simulink library "FuelSystemLibrary"  (R2014b)
settings: Solver=ode45  SolverMode=SingleTasking  StartTime=0.0  StopTime=10.0  RelTol=1e-3
undefined symbols (not defined in the file): BooleanOff, BooleanOn, BoolThreshold, BowserOnPressure, CouplingOffPressure, CouplingOnPressure, DefaultTemp, DiffuserResistance, DiscreteSwitchOff, DiscreteSwitchOn, DiscreteSwitchThreshold, FloatingPressure, FlowNoOverride, FspSamplingPeriod, FuelSpecificHeatCapacity, g, InfiniteFlow, InfiniteMass, InfiniteResistance, InfiniteTime, InfiniteVolume, kpl2kpm3, MaxAValue, MaxBValue, MeterNoReset, MinAValue, MinBValue, NearZeroMass, NearZeroTime, NoError, NominalAValue, NominalBValue, NonRetResistance, NoReset, NullBasePress, PerCycle2PerSec, PerSec2PerCycle, PipeDisconnected, PipeResistance, PumpOnTime, TankFixedMassError, TankInletResistance, TankInstPortStartOffset, TankNoReset, TypicalFuelDensity, ValveClosedPosition, ValveOnResistance, ValveOpenPosition, ValveOpenTime
libraries: FuelSystemLibrary x251, WrightSolverLib x50, simulink x1
(part 1 of 4)
settings Model: ExtModeAutoUpdateStatusClock=off  Creator=SWright2  LastModifiedBy=sj3-wright

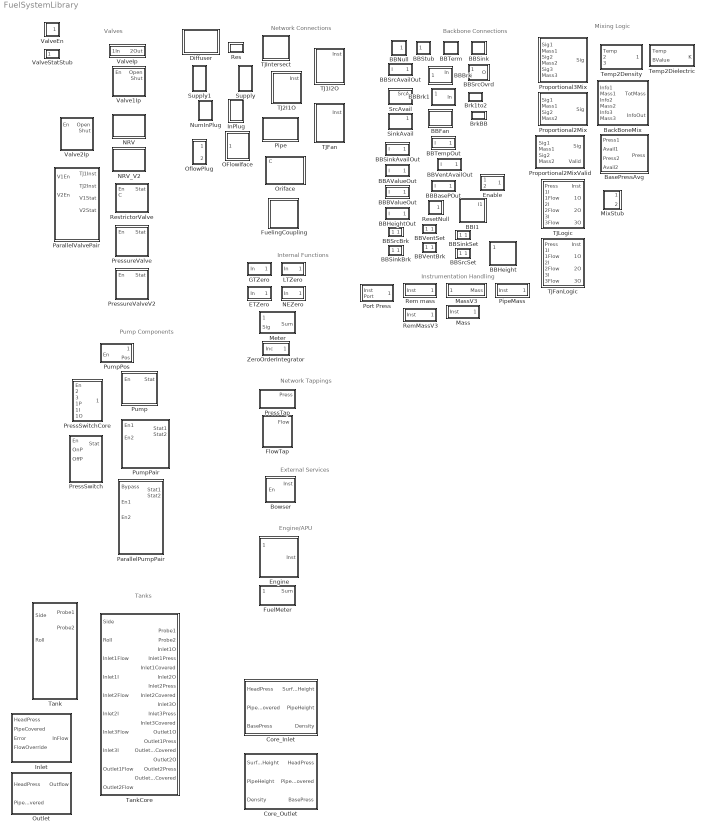
== system FuelSystemLibrary ==
  note: Network Tappings
  note: Network Connections
  note: Valves
  note: Internal Functions
  note: Mixing Logic
  note: External Services
  note: Pump Components
  note: Tanks
  note: Engine/APU
  note: Backbone Connections
  note: Instrumentation Handling
  BBAValueOut : Subsystem
  BBBValueOut : Subsystem
  BBBasePOut : Subsystem
  BBBrk : Subsystem
  BBBrk1 : Subsystem
  BBFan : Subsystem
  BBHeight : Subsystem
  BBHeightOut : Subsystem
  BBI1 : Subsystem
  BBNull : Subsystem
  BBSink : Subsystem
  BBSinkAvailOut : Subsystem
  BBSinkBrk : Subsystem
  BBSinkSet : Subsystem
  BBSrcAvailOut : Subsystem
  BBSrcBrk : Subsystem
  BBSrcOvrd : Subsystem
  BBSrcSet : Subsystem
  BBStub : Subsystem
  BBTempOut : Subsystem
  BBTerm : Subsystem
  BBVentAvailOut : Subsystem
  BBVentBrk : Subsystem
  BBVentSet : Subsystem
  BackBoneMix : Subsystem  RTWFcnName=BackBoneMix  RTWFileName=BackBoneMix
      settings: RTWFcnNameOpts=User specified  RTWFileNameOpts=User specified
  BasePressAvg : Subsystem
  Bowser : Subsystem
  Brk1to2 : Subsystem
  BrkBB : Subsystem
  Core_Inlet : Subsystem
  Core_Outlet : Subsystem
  Diffuser : Subsystem
  ETZero : Subsystem
  Enable : Subsystem
  Engine : Subsystem
  FlowTap : Subsystem
  FuelMeter : Subsystem
  FuelingCoupling : Subsystem
  GTZero : Subsystem  TreatAsAtomicUnit=on
  InPlug : Subsystem
  Inlet : Subsystem  mask{TankInletResistance=TankInletResistance}
      mask init:
      | InfiniteResistance = -999.0;
  LTZero : Subsystem  TreatAsAtomicUnit=on
  Mass : Subsystem
  MassV3 : Subsystem
  Meter : Subsystem  TreatAsAtomicUnit=on  RTWFcnName=Meter  RTWFileName=Meter
      settings: RTWFcnNameOpts=User specified  RTWFileNameOpts=User specified
  MixStub : Subsystem
  NEZero : Subsystem  TreatAsAtomicUnit=on
  NRV : Subsystem
  NRV_V2 : Subsystem
  NumInPlug : Subsystem
  OFlowIface : Subsystem
  OflowPlug : Subsystem
  Oriface : Subsystem
  Outlet : Subsystem
  ParallelPumpPair : Subsystem
  ParallelValvePair : Subsystem
  Pipe : Subsystem
  PipeMass : Subsystem
  Port Press : Subsystem  TreatAsAtomicUnit=on  RTWFcnName=PortPressure  RTWFileName=PortPressure
      settings: RTWFcnNameOpts=User specified  RTWFileNameOpts=User specified
  PressSwitch : Subsystem
  PressSwitchCore : Subsystem  TreatAsAtomicUnit=on  RTWFcnName=PressSwitchCore  RTWFileName=PressSwitchCore
      settings: RTWFcnNameOpts=User specified  RTWFileNameOpts=User specified
  PressTap : Subsystem
  PressureValve : Subsystem
  PressureValveV2 : Subsystem
  Proportional2Mix : Subsystem  RTWFcnName=Proportional2Mix  RTWFileName=Proportional2Mix
      settings: RTWFcnNameOpts=User specified  RTWFileNameOpts=User specified
  Proportional2MixValid : Subsystem  RTWFcnName=Proportional2MixValid  RTWFileName=Proportional2MixValid
      settings: RTWFcnNameOpts=User specified  RTWFileNameOpts=User specified
  Proportional3Mix : Subsystem  RTWFcnName=Proportional3Mix  RTWFileName=Proportional3Mix
      settings: RTWFcnNameOpts=User specified  RTWFileNameOpts=User specified
  Pump : Subsystem
  PumpPair : Subsystem
  PumpPos : Subsystem  TreatAsAtomicUnit=on
  Rem mass : Subsystem
  RemMassV3 : Subsystem
  Res : Subsystem
  ResetNull : Subsystem
  RestrictorValve : Subsystem
  SinkAvail : Subsystem
  SrcAvail : Subsystem
  Supply : Subsystem
  Supply1 : Subsystem
  TJ1I2O : Subsystem
  TJ2I1O : Subsystem
  TJFan : Subsystem
  TJFanLogic : Subsystem
  TJIntersect : Subsystem
  TJLogic : Subsystem
  Tank : Subsystem
  TankCore : Subsystem
      settings: RTWSystemCode=Nonreusable function
  Temp2Density : Subsystem  TreatAsAtomicUnit=on  RTWFcnName=Temp2Density  RTWFileName=Temp2Density
      settings: RTWFcnNameOpts=User specified  RTWFileNameOpts=User specified
  Temp2Dielectric : Subsystem  TreatAsAtomicUnit=on  RTWFcnName=Temp2Dielectric  RTWFileName=Temp2Dielectric
      settings: RTWFcnNameOpts=User specified  RTWFileNameOpts=User specified
  Valve1Ip : Subsystem
  Valve2Ip : Subsystem
  ValveEn : Subsystem  TreatAsAtomicUnit=on  RTWFcnName=ValveEn
      settings: RTWFcnNameOpts=User specified
  ValveIp : Subsystem
  ValveStatStub : Subsystem
  ZeroOrderIntegrator : Subsystem  TreatAsAtomicUnit=on

== system FuelSystemLibrary/BBAValueOut ==
  note: BBAValueOut - Block to seperate Flow A Value form Backbone Network
      |
      | Revision History -
      | Issue 1.0 - ?? - SW - Initial Issue
      | Issue 1.1 - 28th October 2005 - DR - Added to FSP Generic Library
      | Issue 1.2 - 16th December 2008 - SW - SinkAvailable added
  I : Inport
  Demux1 : Demux  Outputs=[1 1 1 1 1 1 1 1]
  Terminator{1..7} (7 alike) : Terminator
  AVal : Outport
  wires:
  I/1 -> Demux1/1
  Demux1/5 -> Terminator6/1  "SrcAvailable"
  Demux1/2 -> Terminator4/1  "Temp"
  Demux1/1 -> Terminator3/1  "BasePress"
  Demux1/3 -> AVal/1  "AValue"
  Demux1/4 -> Terminator5/1  "BValue"
  Demux1/6 -> Terminator1/1  "SinkAvailable"
  Demux1/7 -> Terminator2/1  "VentAvailable"
  Demux1/8 -> Terminator7/1  "Height"

== system FuelSystemLibrary/BBBValueOut ==
  note: BBBValueOut - Block to seperate Flow B Value form Backbone Network
      |
      | Revision History -
      | Issue 1.0 - ?? - SW - Initial Issue
      | Issue 1.1 - 28th October 2005 - DR - Added to FSP Generic Library
      | Issue 1.2 - 16th December 2008 - SW - SinkAvailable added
  I : Inport
  Demux1 : Demux  Outputs=[1 1 1 1 1 1 1 1]
  Terminator{1..7} (7 alike) : Terminator
  BVal : Outport
  wires:
  I/1 -> Demux1/1
  Demux1/5 -> Terminator6/1  "SrcAvailable"
  Demux1/2 -> Terminator4/1  "Temp"
  Demux1/1 -> Terminator3/1  "BasePress"
  Demux1/3 -> Terminator5/1  "AValue"
  Demux1/4 -> BVal/1  "BValue"
  Demux1/6 -> Terminator1/1  "SinkAvailable"
  Demux1/7 -> Terminator2/1  "VentAvailable"
  Demux1/8 -> Terminator7/1  "Height"

== system FuelSystemLibrary/BBBasePOut ==
  note: BBBasePOut - Block to seperate Base Pressure
      | signal from the Backbone Network
      |
      | Revision History -
      | Issue 1.0 - ?? - SW - Initial Issue
      | Issue 1.1 - 28th October 2005 - DR - Added to FSP Generic Library
      | Issue 1.2 - 16th December 2008 - SW - SinkAvailable added
  I : Inport
  Demux1 : Demux  Outputs=[1 1 1 1 1 1 1 1]
  Terminator{1..7} (7 alike) : Terminator
  Press : Outport
  wires:
  I/1 -> Demux1/1
  Demux1/2 -> Terminator3/1  "Temp"
  Demux1/1 -> Press/1  "BasePress"
  Demux1/3 -> Terminator5/1  "AValue"
  Demux1/4 -> Terminator4/1  "BValue"
  Demux1/5 -> Terminator1/1  "SrcAvailable"
  Demux1/6 -> Terminator2/1  "SinkAvailable"
  Demux1/7 -> Terminator6/1  "VentAvailable"
  Demux1/8 -> Terminator7/1  "Height"

== system FuelSystemLibrary/BBBrk ==
  In : Inport
  Two-Way Connection1 : TwoWayConnection
  BB : PMIOPort  Tag=PMCPort  Port=1  Side=Left
  Out : Outport
  wires:
  Two-Way Connection1/1 -> Out/1
  In/1 -> Two-Way Connection1/1
  connections:
  BB/RConn1 -- Two-Way Connection1/RConn1

== system FuelSystemLibrary/BBBrk1 ==
  In : Inport
  Two-Way Connection1 : TwoWayConnection
  BB : PMIOPort  Tag=PMCPort  Port=1  Side=Right
  Out : Outport
  wires:
  In/1 -> Two-Way Connection1/1
  Two-Way Connection1/1 -> Out/1
  connections:
  BB/RConn1 -- Two-Way Connection1/RConn1

== system FuelSystemLibrary/BBFan ==
  BBBrk1 : FuelSystemLibrary/BBBrk1
  BBBrk2 : FuelSystemLibrary/BBBrk1
  BBBrk3 : FuelSystemLibrary/BBBrk1
  BBNull : FuelSystemLibrary/BBNull
  BBStub : FuelSystemLibrary/BBStub
  BBStub1 : FuelSystemLibrary/BBStub
  In : PMIOPort  Tag=PMCPort  Port=1  Side=Left
  Out1 : PMIOPort  Tag=PMCPort  Port=2  Side=Right
  Out2 : PMIOPort  Tag=PMCPort  Port=3  Side=Right
  wires:
  BBBrk3/1 -> BBStub1/1
  BBBrk2/1 -> BBStub/1
  BBNull/1 -> BBBrk1/1
  BBBrk1/1 -> BBBrk3/1, BBBrk2/1
  connections:
  BBBrk3/RConn1 -- Out2/RConn1
  BBBrk2/RConn1 -- Out1/RConn1
  In/RConn1 -- BBBrk1/RConn1

== system FuelSystemLibrary/BBHeight ==
  note: Insert height at this point
  Height : Inport
  BBBrk : FuelSystemLibrary/BBBrk
  BBBrk1 : FuelSystemLibrary/BBBrk1
  Demux1 : Demux  Outputs=[1 1 1 1 1 1 1 1]
  Demux3 : Demux  Outputs=[1 1 1 1 1 1 1 1]
  Mux1 : Mux  Inputs=[1 1 1 1 1 1 1 1]
  Mux3 : Mux  Inputs=[1 1 1 1 1 1 1 1]
  Terminator : Terminator
  Terminator1 : Terminator
  BB1 : PMIOPort  Tag=PMCPort  Port=1  Side=Left
  BB2 : PMIOPort  Tag=PMCPort  Port=2  Side=Right
  wires:
  BBBrk/1 -> Demux1/1
  BBBrk1/1 -> Demux3/1
  [Height] -> Mux3/8
  Demux3/1 -> Mux3/1  "BasePress"
  Demux3/2 -> Mux3/2  "Temp"
  Demux3/3 -> Mux3/3  "AValue"
  Demux3/4 -> Mux3/4  "BValue"
  Demux3/5 -> Mux3/5  "SrcAvailable"
  Demux3/6 -> Mux3/6  "SinkAvailable"
  Demux3/8 -> Terminator/1  "Height"
  Demux3/7 -> Mux3/7  "VentAvailable"
  Mux3/1 -> BBBrk/1
  Demux1/1 -> Mux1/1  "BasePress"
  Demux1/2 -> Mux1/2  "Temp"
  Demux1/3 -> Mux1/3  "AValue"
  Demux1/4 -> Mux1/4  "BValue"
  Demux1/5 -> Mux1/5  "SrcAvailable"
  Demux1/6 -> Mux1/6  "SinkAvailable"
  Demux1/8 -> Terminator1/1  "Height"
  Demux1/7 -> Mux1/7  "VentAvailable"
  Height/1 -> [Height]
  [Height] -> Mux1/8
  Mux1/1 -> BBBrk1/1
  connections:
  BB1/RConn1 -- BBBrk1/RConn1
  BB2/RConn1 -- BBBrk/LConn1

== system FuelSystemLibrary/BBHeightOut ==
  note: BBHeightOut - Block to seperate Height Value form Backbone Network
      |
      | Revision History -
      | Issue 1.0 - 18th Mayt 2009 - SW - Initial Issue
  I : Inport
  Demux1 : Demux  Outputs=[1 1 1 1 1 1 1 1]
  Terminator{1..6,8} (7 alike) : Terminator
  Hght : Outport
  wires:
  I/1 -> Demux1/1
  Demux1/5 -> Terminator6/1  "SrcAvailable"
  Demux1/2 -> Terminator4/1  "Temp"
  Demux1/1 -> Terminator3/1  "BasePress"
  Demux1/3 -> Terminator5/1  "AValue"
  Demux1/4 -> Terminator8/1  "BValue"
  Demux1/6 -> Terminator1/1  "SinkAvailable"
  Demux1/7 -> Terminator2/1  "VentAvailable"
  Demux1/8 -> Hght/1  "Height"

== system FuelSystemLibrary/BBI1 ==
  note: Extract the inbound signal from port1
  BBBrk : FuelSystemLibrary/BBBrk
  BBBrk1 : FuelSystemLibrary/BBBrk1
  BB1 : PMIOPort  Tag=PMCPort  Port=1  Side=Left
  BB2 : PMIOPort  Tag=PMCPort  Port=2  Side=Right
  I1 : Outport
  wires:
  BBBrk1/1 -> I1/1, BBBrk/1
  BBBrk/1 -> BBBrk1/1
  connections:
  BB1/RConn1 -- BBBrk1/RConn1
  BBBrk/LConn1 -- BB2/RConn1

== system FuelSystemLibrary/BBNull ==
  note: BBNull
      |
      | Revision History -
      | Issue 1.0 - ?? - SW - Initial Issue
      | Issue 1.1 - 28th October 2005 - DR - Added to FSP Generic Library
      | Issue 1.2 - 7th July 2009 - SW - New elements added
  Constant1 : Constant  Value=DefaultTemp
  Constant{2,4..6} (4 alike) : Constant  Value=0
  Constant3 : Constant  Value=NullBasePress
  Constant8 : Constant  Value=NominalAValue
  Constant9 : Constant  Value=NominalBValue
  Mux : Mux  Inputs=[1 1 1 1 1 1 1 1]
  Nul : Outport
  wires:
  Constant1/1 -> Mux/2  "Temp"
  Constant3/1 -> Mux/1  "BasePress"
  Constant2/1 -> Mux/5  "SrcAvailable"
  Mux/1 -> Nul/1
  Constant8/1 -> Mux/3  "AValue"
  Constant9/1 -> Mux/4  "BValue"
  Constant4/1 -> Mux/6  "SinkAvailable"
  Constant5/1 -> Mux/7  "VentAvailable"
  Constant6/1 -> Mux/8  "Height"

== system FuelSystemLibrary/BBSink ==
  note: BBTerminator
      |
      | Revision History -
      | Issue 1.0 - 4th April 2011 - SW - Initial Issue
  BBBrk1 : FuelSystemLibrary/BBBrk
  BBBrk2 : FuelSystemLibrary/BBBrk1
  BBSinkSet : FuelSystemLibrary/BBSinkSet
  BBTerm : FuelSystemLibrary/BBTerm
  BB : PMIOPort  Tag=PMCPort  Port=1  Side=Left
  wires:
  BBBrk2/1 -> BBBrk1/1
  BBSinkSet/1 -> BBBrk2/1
  BBBrk1/1 -> BBSinkSet/1
  connections:
  BB/RConn1 -- BBBrk2/RConn1
  BBBrk1/LConn1 -- BBTerm/LConn1

== system FuelSystemLibrary/BBSinkAvailOut ==
  I : Inport
  Data Type Conversion : DataTypeConversion  OutDataTypeStr=double
  Demux : Demux  Outputs=[1 1 1 1 1 1 1 1]
  Terminator{1..7} (7 alike) : Terminator
  SinkA : Outport
  wires:
  Demux/6 -> Data Type Conversion/1  "SinkAvailable"
  Demux/4 -> Terminator5/1  "BValue"
  Demux/3 -> Terminator4/1  "AValue"
  Demux/1 -> Terminator2/1  "BasePress"
  Demux/2 -> Terminator3/1  "Temp"
  Demux/5 -> Terminator1/1  "SrcAvailable"
  I/1 -> Demux/1
  Demux/7 -> Terminator6/1  "VentAvailable"
  Demux/8 -> Terminator7/1  "Height"
  Data Type Conversion/1 -> SinkA/1

== system FuelSystemLibrary/BBSinkBrk ==
  note: Break Backbone Sink-Available Signal
  I : Inport
  Constant1 : Constant  Value=0
  Demux3 : Demux  Outputs=8
  Mux3 : Mux  Inputs=8
  Terminator : Terminator
  O : Outport
  wires:
  Demux3/1 -> Mux3/1  "BasePress"
  Demux3/2 -> Mux3/2  "Temp"
  Demux3/3 -> Mux3/3  "AValue"
  Demux3/4 -> Mux3/4  "BValue"
  Demux3/5 -> Mux3/5  "SrcAvailable"
  Constant1/1 -> Mux3/6
  Demux3/6 -> Terminator/1  "SinkAvailable"
  Demux3/8 -> Mux3/8  "Height"
  Demux3/7 -> Mux3/7  "VentAvailable"
  I/1 -> Demux3/1
  Mux3/1 -> O/1

== system FuelSystemLibrary/BBSinkSet ==
  note: Set Backbone Sink-Available Signal
  I : Inport
  Constant8 : Constant
  Demux2 : Demux  Outputs=8
  Mux3 : Mux  Inputs=8
  Terminator : Terminator
  O : Outport
  wires:
  Mux3/1 -> O/1
  Demux2/7 -> Mux3/7  "VentAvailable"
  Demux2/8 -> Mux3/8  "Height"
  Demux2/6 -> Terminator/1  "SinkAvailable"
  Demux2/5 -> Mux3/5  "SrcAvailable"
  Demux2/4 -> Mux3/4  "BValue"
  Demux2/3 -> Mux3/3  "AValue"
  Demux2/2 -> Mux3/2  "Temp"
  Demux2/1 -> Mux3/1  "BasePress"
  I/1 -> Demux2/1
  Constant8/1 -> Mux3/6

== system FuelSystemLibrary/BBSrcAvailOut ==
  note: BBFlowAvailOut - Block to seperate Flow
      | Available signal from the Backbone Network
      |
      | Revision History -
      | Issue 1.0 - ?? - SW - Initial Issue
      | Issue 1.1 - 28th October 2005 - DR - Added to FSP Generic Library
      | Issue 1.2 - 16th December 2008 - SW - SinkAvailable added
  I : Inport
  Data Type Conversion : DataTypeConversion  OutDataTypeStr=double
  Demux : Demux  Outputs=[1 1 1 1 1 1 1 1]
  Terminator{1..7} (7 alike) : Terminator
  SrcA : Outport
  wires:
  I/1 -> Demux/1
  Demux/5 -> Data Type Conversion/1  "SrcAvailable"
  Demux/2 -> Terminator3/1  "Temp"
  Demux/1 -> Terminator2/1  "BasePress"
  Demux/3 -> Terminator4/1  "AValue"
  Demux/4 -> Terminator5/1  "BValue"
  Demux/6 -> Terminator1/1  "SinkAvailable"
  Demux/7 -> Terminator6/1  "VentAvailable"
  Demux/8 -> Terminator7/1  "Height"
  Data Type Conversion/1 -> SrcA/1

== system FuelSystemLibrary/BBSrcBrk ==
  note: Break Backbone Sink-Available Signal
  I : Inport
  Constant1 : Constant  Value=0
  Demux3 : Demux  Outputs=8
  Mux3 : Mux  Inputs=8
  Terminator : Terminator
  O : Outport
  wires:
  Mux3/1 -> O/1
  I/1 -> Demux3/1
  Demux3/7 -> Mux3/7  "VentAvailable"
  Demux3/8 -> Mux3/8  "Height"
  Demux3/6 -> Mux3/6  "SinkAvailable"
  Demux3/5 -> Terminator/1  "SrcAvailable"
  Demux3/4 -> Mux3/4  "BValue"
  Demux3/3 -> Mux3/3  "AValue"
  Demux3/2 -> Mux3/2  "Temp"
  Demux3/1 -> Mux3/1  "BasePress"
  Constant1/1 -> Mux3/5

== system FuelSystemLibrary/BBSrcOvrd ==
  note: Override BB SrcAvailable signal
  Src : Inport
  I : Inport  Port=2
  Demux3 : Demux  Outputs=8
  Mux3 : Mux  Inputs=8
  Terminator : Terminator
  O : Outport
  wires:
  Demux3/1 -> Mux3/1  "BasePress"
  Demux3/2 -> Mux3/2  "Temp"
  Demux3/3 -> Mux3/3  "AValue"
  Demux3/4 -> Mux3/4  "BValue"
  Demux3/5 -> Terminator/1  "SrcAvailable"
  Src/1 -> Mux3/5
  Demux3/6 -> Mux3/6  "SinkAvailable"
  Demux3/8 -> Mux3/8  "Height"
  Demux3/7 -> Mux3/7  "VentAvailable"
  I/1 -> Demux3/1
  Mux3/1 -> O/1

== system FuelSystemLibrary/BBSrcSet ==
  note: Set Backbone Source-Available Signal
  I : Inport
  Constant8 : Constant
  Demux2 : Demux  Outputs=8
  Mux3 : Mux  Inputs=8
  Terminator : Terminator
  O : Outport
  wires:
  I/1 -> Demux2/1
  Demux2/1 -> Mux3/1  "BasePress"
  Demux2/2 -> Mux3/2  "Temp"
  Demux2/3 -> Mux3/3  "AValue"
  Demux2/4 -> Mux3/4  "BValue"
  Demux2/5 -> Terminator/1  "SrcAvailable"
  Demux2/6 -> Mux3/6  "SinkAvailable"
  Demux2/8 -> Mux3/8  "Height"
  Demux2/7 -> Mux3/7  "VentAvailable"
  Mux3/1 -> O/1
  Constant8/1 -> Mux3/5

== system FuelSystemLibrary/BBStub ==
  note: BBStub
      |
      | Revision History -
      | Issue 1.0 - ?? - SW - Initial Issue
      | Issue 1.1 - 28th October 2005 - DR - Added to FSP Generic Library
      | Issue 1.2 - 7th July 2009 - SW - New elements added
  Nul : Inport
  Demux4 : Demux  Outputs=[1 1 1 1 1 1 1 1]
  Terminator{1..8} (8 alike) : Terminator
  wires:
  Demux4/4 -> Terminator5/1  "BValue"
  Demux4/3 -> Terminator3/1  "AValue"
  Demux4/5 -> Terminator6/1  "SrcAvailable"
  Demux4/2 -> Terminator2/1  "Temp"
  Demux4/1 -> Terminator4/1  "BasePress"
  Nul/1 -> Demux4/1
  Demux4/6 -> Terminator1/1  "SinkAvailable"
  Demux4/7 -> Terminator7/1  "VentAvailable"
  Demux4/8 -> Terminator8/1  "Height"

== system FuelSystemLibrary/BBTempOut ==
  note: BBTempOut - Block to seperate Flow
      | Temperature signal from the Backbone Network
      |
      | Revision History -
      | Issue 1.0 - ?? - SW - Initial Issue
      | Issue 1.1 - 28th October 2005 - DR - Added to FSP Generic Library
  I : Inport
  Demux1 : Demux  Outputs=[1 1 1 1 1 1 1 1]
  Terminator{1..7} (7 alike) : Terminator
  Temp : Outport
  wires:
  I/1 -> Demux1/1
  Demux1/5 -> Terminator6/1  "SrcAvailable"
  Demux1/2 -> Temp/1  "Temp"
  Demux1/1 -> Terminator3/1  "BasePress"
  Demux1/3 -> Terminator5/1  "AValue"
  Demux1/4 -> Terminator4/1  "BValue"
  Demux1/6 -> Terminator1/1  "SinkAvailable"
  Demux1/7 -> Terminator2/1  "VentAvailable"
  Demux1/8 -> Terminator7/1  "Height"

== system FuelSystemLibrary/BBTerm ==
  note: BBTerminator
      |
      | Revision History -
      | Issue 1.0 - 1st December 2009 - SW - Initial Issue
  BBBrk : FuelSystemLibrary/BBBrk
  Constant1 : Constant  Value=DefaultTemp
  Constant2 : Constant  Value=0
  Constant3 : Constant  Value=NullBasePress
  Constant4 : Constant  Value=0
  Constant5 : Constant  Value=0
  Constant8 : Constant  Value=NominalAValue
  Constant9 : Constant  Value=NominalBValue
  Demux4 : Demux  Outputs=[1 1 1 1 1 1 1 1]
  Mux : Mux  Inputs=[1 1 1 1 1 1 1 1]
  Terminator{1..7} (7 alike) : Terminator
  Unit Delay2 : UnitDelay  SampleTime=FspSamplingPeriod
  BB : PMIOPort  Tag=PMCPort  Port=1  Side=Left
  wires:
  BBBrk/1 -> Demux4/1
  Mux/1 -> BBBrk/1
  Unit Delay2/1 -> Mux/8  "Height"
  Constant5/1 -> Mux/7  "VentAvailable"
  Constant4/1 -> Mux/6  "SinkAvailable"
  Constant9/1 -> Mux/4  "BValue"
  Constant8/1 -> Mux/3  "AValue"
  Constant2/1 -> Mux/5  "SrcAvailable"
  Constant3/1 -> Mux/1  "BasePress"
  Constant1/1 -> Mux/2  "Temp"
  Demux4/8 -> Unit Delay2/1  "Height"
  Demux4/7 -> Terminator7/1  "VentAvailable"
  Demux4/6 -> Terminator1/1  "SinkAvailable"
  Demux4/1 -> Terminator4/1  "BasePress"
  Demux4/2 -> Terminator2/1  "Temp"
  Demux4/5 -> Terminator6/1  "SrcAvailable"
  Demux4/3 -> Terminator3/1  "AValue"
  Demux4/4 -> Terminator5/1  "BValue"
  connections:
  BB/RConn1 -- BBBrk/LConn1

== system FuelSystemLibrary/BBVentAvailOut ==
  note: BBSinkAvailOut - Block to seperate Flow
      | Available signal from the Backbone Network
      |
      | Revision History -
      | Issue 1.0 - ?? - SW - Initial Issue
      | Issue 1.1 - 28th October 2005 - DR - Added to FSP Generic Library
      | Issue 1.2 - 16th December 2008 - SW - SinkAvailable added
  I : Inport
  Data Type Conversion : DataTypeConversion  OutDataTypeStr=double
  Demux : Demux  Outputs=[1 1 1 1 1 1 1 1]
  Terminator{1..7} (7 alike) : Terminator
  Vent : Outport
  wires:
  Demux/6 -> Terminator6/1  "SinkAvailable"
  Demux/4 -> Terminator5/1  "BValue"
  Demux/3 -> Terminator4/1  "AValue"
  Demux/1 -> Terminator2/1  "BasePress"
  Demux/2 -> Terminator3/1  "Temp"
  Demux/5 -> Terminator1/1  "SrcAvailable"
  I/1 -> Demux/1
  Demux/7 -> Data Type Conversion/1  "VentAvailable"
  Demux/8 -> Terminator7/1  "Height"
  Data Type Conversion/1 -> Vent/1

== system FuelSystemLibrary/BBVentBrk ==
  note: Break Backbone Vent-Available Signal
  I : Inport
  Constant8 : Constant  Value=0
  Demux2 : Demux  Outputs=8
  Mux3 : Mux  Inputs=8
  Terminator : Terminator
  O : Outport
  wires:
  Mux3/1 -> O/1
  Demux2/7 -> Terminator/1  "VentAvailable"
  Constant8/1 -> Mux3/7
  Demux2/8 -> Mux3/8  "Height"
  Demux2/6 -> Mux3/6  "SinkAvailable"
  Demux2/5 -> Mux3/5  "SrcAvailable"
  Demux2/4 -> Mux3/4  "BValue"
  Demux2/3 -> Mux3/3  "AValue"
  Demux2/2 -> Mux3/2  "Temp"
  Demux2/1 -> Mux3/1  "BasePress"
  I/1 -> Demux2/1

== system FuelSystemLibrary/BBVentSet ==
  note: Set Backbone Vent-Available Signal
  I : Inport
  Constant8 : Constant
  Demux2 : Demux  Outputs=8
  Mux3 : Mux  Inputs=8
  Terminator : Terminator
  O : Outport
  wires:
  I/1 -> Demux2/1
  Demux2/1 -> Mux3/1  "BasePress"
  Demux2/2 -> Mux3/2  "Temp"
  Demux2/3 -> Mux3/3  "AValue"
  Demux2/4 -> Mux3/4  "BValue"
  Demux2/5 -> Mux3/5  "SrcAvailable"
  Demux2/6 -> Mux3/6  "SinkAvailable"
  Demux2/8 -> Mux3/8  "Height"
  Constant8/1 -> Mux3/7
  Demux2/7 -> Terminator/1  "VentAvailable"
  Mux3/1 -> O/1

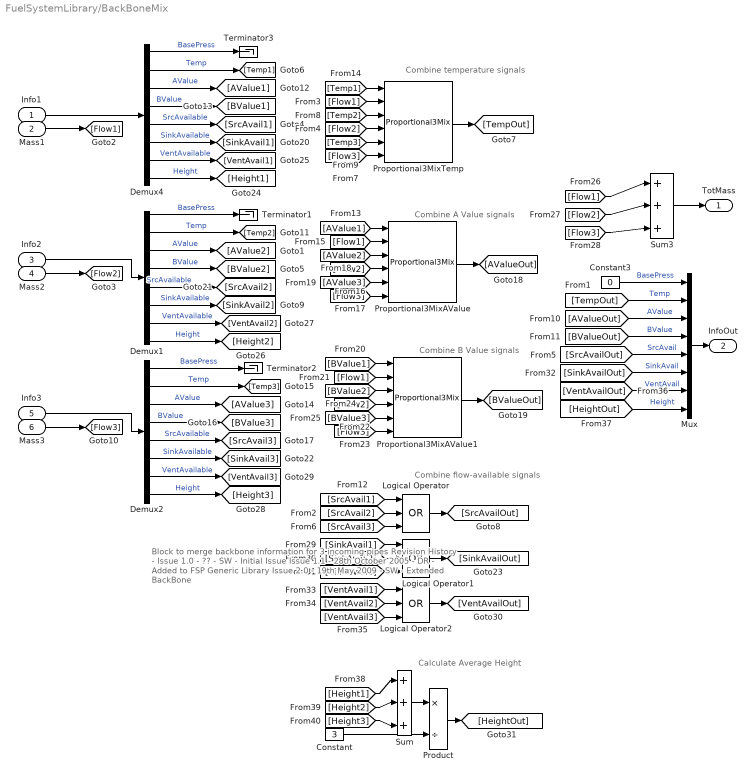
== system FuelSystemLibrary/BackBoneMix ==
  note: Block to merge backbone information for 3 incoming pipes
      |
      | Revision History -
      | Issue 1.0 - ?? - SW - Initial Issue
      | Issue 1.1 - 28th October 2005 - DR - Added to FSP Generic Library
      | Issue 2.0 - 19th May 2009 - SW - Extended BackBone
  note: Combine temperature signals
  note: Combine flow-available signals
  note: Combine A Value signals
  note: Combine B Value signals
  note: Calculate Average Height
  Info1 : Inport
  Mass1 : Inport  Port=2
  Info2 : Inport  Port=3
  Mass2 : Inport  Port=4
  Info3 : Inport  Port=5
  Mass3 : Inport  Port=6
  Constant : Constant  Value=3
  Constant3 : Constant  Value=0
  Demux1 : Demux  Outputs=[1 1 1 1 1 1 1 1]
  Demux2 : Demux  Outputs=[1 1 1 1 1 1 1 1]
  Demux4 : Demux  Outputs=[1 1 1 1 1 1 1 1]
  Logical Operator : Logic  Operator=OR  Inputs=3  AllPortsSameDT=off
  Logical Operator1 : Logic  Operator=OR  Inputs=3  AllPortsSameDT=off
  Logical Operator2 : Logic  Operator=OR  Inputs=3  AllPortsSameDT=off
  Mux : Mux  Inputs=8
  Product : Product  Inputs=*/  SaturateOnIntegerOverflow=on  InputSameDT=on  OutDataTypeStr=Inherit: Same as first input
  Proportional3MixAValue : FuelSystemLibrary/Proportional3Mix
  Proportional3MixAValue1 : FuelSystemLibrary/Proportional3Mix
  Proportional3MixTemp : FuelSystemLibrary/Proportional3Mix
  Sum : Sum  Inputs=|+++  SaturateOnIntegerOverflow=on  InputSameDT=on  OutDataTypeStr=Inherit: Same as first input
  Sum3 : Sum  Inputs=|+++  SaturateOnIntegerOverflow=on
  Terminator1 : Terminator
  Terminator2 : Terminator
  Terminator3 : Terminator
  TotMass : Outport
  InfoOut : Outport  Port=2
  wires:
  Mass1/1 -> [Flow1]
  Mass2/1 -> [Flow2]
  [Temp2] -> Proportional3MixTemp/3
  [Flow2] -> Proportional3MixTemp/4
  [Temp1] -> Proportional3MixTemp/1
  [Flow1] -> Proportional3MixTemp/2
  Mux/1 -> InfoOut/1
  Info1/1 -> Demux4/1
  Proportional3MixTemp/1 -> [TempOut]
  [SrcAvail2] -> Logical Operator/2
  [SrcAvail1] -> Logical Operator/1
  Logical Operator/1 -> [SrcAvailOut]
  Constant3/1 -> Mux/1  "BasePress"
  [TempOut] -> Mux/2  "Temp"
  [SrcAvailOut] -> Mux/5  "SrcAvail"
  Info3/1 -> Demux2/1
  Mass3/1 -> [Flow3]
  [SrcAvail3] -> Logical Operator/3
  [Temp3] -> Proportional3MixTemp/5
  [Flow3] -> Proportional3MixTemp/6
  Demux4/1 -> Terminator3/1  "BasePress"
  Demux4/2 -> [Temp1]  "Temp"
  Demux4/5 -> [SrcAvail1]  "SrcAvailable"
  Demux4/3 -> [AValue1]  "AValue"
  Demux4/4 -> [BValue1]  "BValue"
  Info2/1 -> Demux1/1
  Demux1/1 -> Terminator1/1  "BasePress"
  Demux1/2 -> [Temp2]  "Temp"
  Demux1/3 -> [AValue2]  "AValue"
  Demux1/4 -> [BValue2]  "BValue"
  Demux2/1 -> Terminator2/1  "BasePress"
  Demux2/2 -> [Temp3]  "Temp"
  Demux2/3 -> [AValue3]  "AValue"
  Demux2/4 -> [BValue3]  "BValue"
  [AValueOut] -> Mux/3  "AValue"
  [BValueOut] -> Mux/4  "BValue"
  [AValue2] -> Proportional3MixAValue/3
  [Flow2] -> Proportional3MixAValue/4
  [AValue1] -> Proportional3MixAValue/1
  [Flow1] -> Proportional3MixAValue/2
  Proportional3MixAValue/1 -> [AValueOut]
  [AValue3] -> Proportional3MixAValue/5
  [Flow3] -> Proportional3MixAValue/6
  [BValue2] -> Proportional3MixAValue1/3
  [Flow2] -> Proportional3MixAValue1/4
  [BValue1] -> Proportional3MixAValue1/1
  [Flow1] -> Proportional3MixAValue1/2
  Proportional3MixAValue1/1 -> [BValueOut]
  [BValue3] -> Proportional3MixAValue1/5
  [Flow3] -> Proportional3MixAValue1/6
  [Flow1] -> Sum3/1
  [Flow2] -> Sum3/2
  [Flow3] -> Sum3/3
  Sum3/1 -> TotMass/1
  Demux4/6 -> [SinkAvail1]  "SinkAvailable"
  Demux1/5 -> [SrcAvail2]  "SrcAvailable"
  Demux1/6 -> [SinkAvail2]  "SinkAvailable"
  Demux2/5 -> [SrcAvail3]  "SrcAvailable"
  Demux2/6 -> [SinkAvail3]  "SinkAvailable"
  [SinkAvail2] -> Logical Operator1/2
  [SinkAvail1] -> Logical Operator1/1
  Logical Operator1/1 -> [SinkAvailOut]
  [SinkAvail3] -> Logical Operator1/3
  [SinkAvailOut] -> Mux/6  "SinkAvail"
  Demux4/7 -> [VentAvail1]  "VentAvailable"
  Demux4/8 -> [Height1]  "Height"
  Demux1/7 -> [VentAvail2]  "VentAvailable"
  Demux1/8 -> [Height2]  "Height"
  Demux2/7 -> [VentAvail3]  "VentAvailable"
  Demux2/8 -> [Height3]  "Height"
  [VentAvail2] -> Logical Operator2/2
  [VentAvail1] -> Logical Operator2/1
  Logical Operator2/1 -> [VentAvailOut]
  [VentAvail3] -> Logical Operator2/3
  [VentAvailOut] -> Mux/7  "VentAvail"
  [HeightOut] -> Mux/8  "Height"
  [Height1] -> Sum/1
  [Height2] -> Sum/2
  [Height3] -> Sum/3
  Sum/1 -> Product/1
  Product/1 -> [HeightOut]
  Constant/1 -> Product/2

== system FuelSystemLibrary/BasePressAvg ==
  note: Average incoming pressures, ignoring non-connected inlets
      |
      | Revision History -
      | Issue 1.0 - ?? - SW - Initial Issue
      | Issue 1.1 - 28th October 2005 - DR - Added to FSP Generic Library
  note: Avoid div-by-zero
  Press1 : Inport
  Avail1 : Inport  Port=2
  Press2 : Inport  Port=3
  Avail2 : Inport  Port=4
  Constant : Constant
  ETZero : FuelSystemLibrary/ETZero
  Product : Product  SaturateOnIntegerOverflow=on  InputSameDT=on  OutDataTypeStr=Inherit: Same as first input
  Product1 : Product  SaturateOnIntegerOverflow=on  InputSameDT=on  OutDataTypeStr=Inherit: Same as first input
  Product3 : Product  Inputs=*/  SaturateOnIntegerOverflow=on  InputSameDT=on  OutDataTypeStr=Inherit: Same as first input
  Sum : Sum  Inputs=|++  SaturateOnIntegerOverflow=on  InputSameDT=on  OutDataTypeStr=Inherit: Same as first input
  Sum1 : Sum  Inputs=|++  SaturateOnIntegerOverflow=on  InputSameDT=on  OutDataTypeStr=Inherit: Same as first input
  Switch : Switch  Threshold=BoolThreshold  SaturateOnIntegerOverflow=on
  Press : Outport
  wires:
  Sum1/1 -> Product3/1
  Product/1 -> Sum1/1
  Product1/1 -> Sum1/2
  Press1/1 -> Product/1
  Avail1/1 -> Product/2, Sum/1
  Avail2/1 -> Product1/2, Sum/2
  Press2/1 -> Product1/1
  Sum/1 -> ETZero/1, Switch/3  "Total"
  ETZero/1 -> Switch/2
  Constant/1 -> Switch/1
  Switch/1 -> Product3/2
  Product3/1 -> Press/1

== system FuelSystemLibrary/Bowser ==
  note: Flow always available from bowser
  note: Pump modelled as
      | effort source
  note: Enable valve if bowser enabled
  En : Inport
  BBBrk3 : FuelSystemLibrary/BBBrk
  BBNull : FuelSystemLibrary/BBNull
  BBSrcOvrd : FuelSystemLibrary/BBSrcOvrd
  BBStub1 : FuelSystemLibrary/BBStub
  Constant : Constant  Value=MeterNoReset
  Constant1 : Constant  Value=BooleanOn
  Constant12 : Constant  Value=FlowNoOverride
  Constant2 : Constant  Value=MeterNoReset
  Constant3 : Constant  Value=BowserOnPressure
  FuelMeter : Subsystem
  Mux1 : Mux  Inputs=2
  NEZero : FuelSystemLibrary/NEZero
  Subsystem4 : Subsystem
  Term : WrightSolverLib/Term
  V : WrightSolverLib/V
  Valve1Ip : FuelSystemLibrary/Valve1Ip
  P : PMIOPort  Tag=PMCPort  Port=1  Side=Right
  BB : PMIOPort  Tag=PMCPort  Port=2  Side=Right
  Inst : Outport
  wires:
  Mux1/1 -> Inst/1
  FuelMeter/2(DefuelSum) -> Mux1/2
  FuelMeter/1(RefuelSum) -> Mux1/1
  Constant/1 -> FuelMeter/1(RefuelReset)
  Constant2/1 -> FuelMeter/2(DefuelReset)
  En/1 -> NEZero/1
  Valve1Ip/1 -> Subsystem4/1(1)
  Constant12/1 -> V/3, V/2
  NEZero/1 -> Valve1Ip/1
  BBSrcOvrd/1 -> BBBrk3/1
  BBBrk3/1 -> BBStub1/1
  BBNull/1 -> BBSrcOvrd/2
  Constant1/1 -> BBSrcOvrd/1
  Constant3/1 -> V/1
  Valve1Ip/2 -> Subsystem4/2(2)
  connections:
  FuelMeter/RConn1 -- P/RConn1
  Valve1Ip/RConn1 -- FuelMeter/LConn1
  Valve1Ip/RConn2 -- BB/RConn1
  V/RConn1 -- Valve1Ip/LConn1
  Term/RConn1 -- V/LConn1
  BBBrk3/LConn1 -- Valve1Ip/LConn2

== system FuelSystemLibrary/Brk1to2 ==
  BBBrk : FuelSystemLibrary/BBBrk
  BBBrk2 : FuelSystemLibrary/BBBrk1
  Delay : UnitDelay  InitialCondition=[NullBasePress DefaultTemp NominalAValue NominalBValue 0 0 0 0]  SampleTime=FspSamplingPeriod
  1 : PMIOPort  Tag=PMCPort  Port=1  Side=Left
  2 : PMIOPort  Tag=PMCPort  Port=2  Side=Right
  wires:
  BBBrk/1 -> BBBrk2/1
  BBBrk2/1 -> Delay/1
  Delay/1 -> BBBrk/1
  connections:
  1/RConn1 -- BBBrk2/RConn1
  BBBrk/LConn1 -- 2/RConn1

== system FuelSystemLibrary/BrkBB ==
  BBBrk1 : FuelSystemLibrary/BBBrk1
  BBBrk2 : FuelSystemLibrary/BBBrk
  Delay : UnitDelay  InitialCondition=[NullBasePress DefaultTemp NominalAValue NominalBValue 0 0 0 0]  SampleTime=FspSamplingPeriod
  Delay1 : UnitDelay  InitialCondition=[NullBasePress DefaultTemp NominalAValue NominalBValue 0 0 0 0]  SampleTime=FspSamplingPeriod
  1 : PMIOPort  Tag=PMCPort  Port=1  Side=Left
  2 : PMIOPort  Tag=PMCPort  Port=2  Side=Right
  wires:
  Delay/1 -> BBBrk2/1
  BBBrk1/1 -> Delay/1
  BBBrk2/1 -> Delay1/1
  Delay1/1 -> BBBrk1/1
  connections:
  BBBrk2/LConn1 -- 2/RConn1
  1/RConn1 -- BBBrk1/RConn1

== system FuelSystemLibrary/Core_Inlet ==
  note: Calculate head pressure from surface height - pgh
  note: Still get head pressure due to whole
      | pipe height if level goes below pipes
  note: Decide if pipe is covered
  note: No inlet outflow if level
      | is below the pipe level
  note: No inlet outflow if pipe
      | is disconnected
  note: Calculate base pressure from pipe height - pgh
  SurfaceHeight : Inport
  PipeHeight : Inport  Port=2
  Density : Inport  Port=3
  Constant1 : Constant  Value=PipeDisconnected
  Constant2 : Constant  Value=g
  Constant4 : Constant  Value=g
  Data Type Conversion : DataTypeConversion  OutDataTypeStr=double
  Logical Operator : Logic  AllPortsSameDT=off
  Product1 : Product  Inputs=3  SaturateOnIntegerOverflow=on  InputSameDT=on  OutDataTypeStr=Inherit: Same as first input
  Product2 : Product  Inputs=3  SaturateOnIntegerOverflow=on  InputSameDT=on  OutDataTypeStr=Inherit: Same as first input
  Relational Operator1 : RelationalOperator  Operator=>  InputSameDT=on
  Relational Operator2 : RelationalOperator  Operator=~=  InputSameDT=on
  Switch1 : Switch  Threshold=BoolThreshold  SaturateOnIntegerOverflow=on  InputSameDT=on
  HeadPress : Outport
  PipeCovered : Outport  Port=2
  BasePress : Outport  Port=3
  wires:
  [FuelDensity] -> Product2/1
  Density/1 -> [FuelDensity]
  PipeHeight/1 -> [PipeHeight]
  SurfaceHeight/1 -> [SurfaceHeight]
  [SurfaceHeight] -> Switch1/1
  [PipeHeight] -> Switch1/3
  Constant4/1 -> Product2/2
  [Covered] -> Switch1/2
  Switch1/1 -> Product2/3
  Product2/1 -> HeadPress/1
  Relational Operator1/1 -> Logical Operator/1
  [SurfaceHeight] -> Relational Operator1/1
  [PipeHeight] -> Relational Operator1/2
  [Covered] -> Data Type Conversion/1
  [PipeHeight] -> Relational Operator2/1
  Constant1/1 -> Relational Operator2/2
  Relational Operator2/1 -> Logical Operator/2
  Logical Operator/1 -> [Covered]
  [FuelDensity] -> Product1/1
  [PipeHeight] -> Product1/3
  Constant2/1 -> Product1/2
  Product1/1 -> BasePress/1
  Data Type Conversion/1 -> PipeCovered/1

== system FuelSystemLibrary/Core_Outlet ==
  note: Decide if pipe is covered
  note: Still get head pressure due to whole
      | pipe height if level goes below pipes
  note: Calculate head pressure from surface height - pgh
  note: No inlet outflow if pipe
      | is disconnected
  note: No inlet outflow if level
      | is below the pipe level
  note: Calculate base pressure from pipe height - pgh
  SurfaceHeight : Inport
  PipeHeight : Inport  Port=2
  Density : Inport  Port=3
  Constant1 : Constant  Value=PipeDisconnected
  Constant2 : Constant  Value=g
  Constant4 : Constant  Value=g
  Data Type Conversion : DataTypeConversion  OutDataTypeStr=double
  Logical Operator : Logic  AllPortsSameDT=off
  Product1 : Product  Inputs=3  SaturateOnIntegerOverflow=on  InputSameDT=on  OutDataTypeStr=Inherit: Same as first input
  Product2 : Product  Inputs=3  SaturateOnIntegerOverflow=on  InputSameDT=on  OutDataTypeStr=Inherit: Same as first input
  Relational Operator1 : RelationalOperator  Operator=>  InputSameDT=on
  Relational Operator2 : RelationalOperator  Operator=~=  InputSameDT=on
  Switch1 : Switch  Threshold=BoolThreshold  SaturateOnIntegerOverflow=on  InputSameDT=on
  HeadPress : Outport
  PipeCovered : Outport  Port=2
  BasePress : Outport  Port=3
  wires:
  Logical Operator/1 -> [Covered]
  Switch1/1 -> Product2/3
  [Covered] -> Switch1/2
  Constant4/1 -> Product2/2
  [SurfaceHeight] -> Switch1/1
  SurfaceHeight/1 -> [SurfaceHeight]
  PipeHeight/1 -> [PipeHeight]
  Density/1 -> [FuelDensity]
  [FuelDensity] -> Product2/1
  [Covered] -> Data Type Conversion/1
  [PipeHeight] -> Switch1/3
  Product2/1 -> HeadPress/1
  Relational Operator2/1 -> Logical Operator/2
  Constant1/1 -> Relational Operator2/2
  [PipeHeight] -> Relational Operator2/1
  [PipeHeight] -> Relational Operator1/2
  [SurfaceHeight] -> Relational Operator1/1
  Relational Operator1/1 -> Logical Operator/1
  Constant2/1 -> Product1/2
  [FuelDensity] -> Product1/1
  [PipeHeight] -> Product1/3
  Product1/1 -> BasePress/1
  Data Type Conversion/1 -> PipeCovered/1

== system FuelSystemLibrary/Diffuser ==
  Constant1 : Constant  Value=DiffuserResistance
  Res : WrightSolverLib/Res
  Terminator8 : Terminator
  1P : PMIOPort  Tag=PMCPort  Port=1  Side=Left
  1BB : PMIOPort  Tag=PMCPort  Port=2  Side=Left
  2P : PMIOPort  Tag=PMCPort  Port=3  Side=Right
  2BB : PMIOPort  Tag=PMCPort  Port=4  Side=Right
  wires:
  Constant1/1 -> Res/1
  Res/1 -> Terminator8/1
  connections:
  1BB/RConn1 -- 2BB/RConn1
  1P/RConn1 -- Res/LConn1
  Res/RConn1 -- 2P/RConn1

== system FuelSystemLibrary/ETZero ==
  note: ETZero
      |
      | Revision History -
      | Issue 1.0 - ?? - SW - Initial Issue
      | Issue 1.1 - 28th October 2005 - DR - Added to FSP Generic Library
  In : Inport
  Constant : Constant  Value=0
  Relational Operator : RelationalOperator  Operator===  InputSameDT=on
  =0 : Outport
  wires:
  In/1 -> Relational Operator/1
  Constant/1 -> Relational Operator/2
  Relational Operator/1 -> =0/1

== system FuelSystemLibrary/Enable ==
  Sig : Inport
  En : Inport  Port=2
  Constant8 : Constant  Value=0
  Switch4 : Switch  Threshold=DiscreteSwitchThreshold  SaturateOnIntegerOverflow=on  InputSameDT=on
  Out : Outport
  wires:
  Switch4/1 -> Out/1
  En/1 -> Switch4/2
  Constant8/1 -> Switch4/3
  Sig/1 -> Switch4/1

== system FuelSystemLibrary/Engine ==
  note: Engine is 0.5m
      | below feed pipes
  note: Pressure due to level
  Throttle : Inport  OutDataTypeStr=double
  BBBrk1 : FuelSystemLibrary/BBBrk1
  BBHeightOut : FuelSystemLibrary/BBHeightOut
  Constant1 : Constant  Value=DefaultTemp
  Constant10 : Constant  Value=0.0
  Constant12 : Constant  Value=FlowNoOverride
  Constant2 : Constant  Value=0
  Constant3 : Constant  Value=g
  Constant4 : Constant  Value=0
  Constant5 : Constant  Value=0.5
  Constant6 : Constant
  Constant7 : Constant  Value=TypicalFuelDensity
  Constant8 : Constant  Value=NominalAValue
  Constant9 : Constant  Value=NominalBValue
  Data Type Conversion2 : DataTypeConversion  OutDataTypeStr=double  SaturateOnIntegerOverflow=on  RndMeth=Zero
  FuelMeter : FuelSystemLibrary/FuelMeter
  I : WrightSolverLib/I
  Mux1 : Mux  Inputs=8
  PipePressNEZero1 : FuelSystemLibrary/NEZero
  Prevent -ve demand : Saturate  UpperLimit=InfiniteFlow  LowerLimit=0
  Product3 : Product  Inputs=3  SaturateOnIntegerOverflow=on  InputSameDT=on  OutDataTypeStr=Inherit: Same as first input
  Sum : Sum  Inputs=|+-  SaturateOnIntegerOverflow=on
  Term : WrightSolverLib/Term
  V : WrightSolverLib/V
  P : PMIOPort  Tag=PMCPort  Port=1  Side=Left
  BB : PMIOPort  Tag=PMCPort  Port=2  Side=Left
  Inst : Outport
  wires:
  Mux1/1 -> BBBrk1/1
  BBBrk1/1 -> BBHeightOut/1
  Constant1/1 -> Mux1/2  "Temp"
  Constant4/1 -> Mux1/1  "BasePress"
  Constant2/1 -> Mux1/5  "SrcAvailable"
  Constant8/1 -> Mux1/3  "AValue"
  Constant9/1 -> Mux1/4  "BValue"
  Throttle/1 -> Prevent -ve demand/1  "Throttle"
  FuelMeter/1 -> [FuelBurnt]
  Prevent -ve demand/1 -> PipePressNEZero1/1, I/1
  [DemandOn] -> Mux1/6  "SinkAvailable"
  Constant6/1 -> Mux1/7  "VentAvailable"
  [EngHeight] -> Mux1/8  "Height"
  BBHeightOut/1 -> [Height]
  PipePressNEZero1/1 -> Data Type Conversion2/1
  Data Type Conversion2/1 -> [DemandOn]
  [Height] -> Sum/1
  Constant5/1 -> Sum/2
  Constant7/1 -> Product3/1
  [EngHeight] -> Product3/3
  Constant3/1 -> Product3/2
  Product3/1 -> V/1
  Constant12/1 -> V/2, V/3
  Sum/1 -> [EngHeight]
  Constant10/1 -> FuelMeter/1
  [FuelBurnt] -> Inst/1
  connections:
  BB/RConn1 -- BBBrk1/RConn1
  FuelMeter/RConn1 -- I/LConn1
  P/RConn1 -- FuelMeter/LConn1
  V/RConn1 -- I/RConn1
  Term/RConn1 -- V/LConn1

== system FuelSystemLibrary/FlowTap ==
  note: FlowTap
      |
      | Revision History -
      | Issue 1.0 - ?? - SW - Initial Issue
      | Issue 1.1 - 28th October 2005 - DR - Added to FSP Generic Library
  note: Measure flow in network line
  I Tap : WrightSolverLib/I Tap
  1P : PMIOPort  Tag=PMCPort  Port=1  Side=Left
  1BB : PMIOPort  Tag=PMCPort  Port=2  Side=Left
  2P : PMIOPort  Tag=PMCPort  Port=3  Side=Right
  2BB : PMIOPort  Tag=PMCPort  Port=4  Side=Right
  Flow : Outport
  wires:
  I Tap/1 -> Flow/1
  connections:
  1BB/RConn1 -- 2BB/RConn1
  I Tap/RConn1 -- 2P/RConn1
  1P/RConn1 -- I Tap/LConn1

== system FuelSystemLibrary/FuelMeter ==
  note: Fuel meter
      |
      | Revision History -
      | Issue 1.0 - ?? - SW - Initial Issue
      | Issue 1.1 - 28th October 2005 - DR - Added to FSP Generic Library
  Reset : Inport
  I Tap : WrightSolverLib/I Tap
  Meter : FuelSystemLibrary/Meter
  1P : PMIOPort  Tag=PMCPort  Port=1  Side=Left
  2P : PMIOPort  Tag=PMCPort  Port=2  Side=Right
  Sum : Outport
  wires:
  Reset/1 -> Meter/1
  I Tap/1 -> Meter/2
  Meter/1 -> Sum/1
  connections:
  I Tap/RConn1 -- 2P/RConn1
  1P/RConn1 -- I Tap/LConn1

== system FuelSystemLibrary/FuelingCoupling ==
  note: FuelingCoupling: Simulation of refuel/defuel coupling
      |
      | Change History:
      | Issue 1.0: 27/10/2004: Fix to cross-pressure calculation bug - Sw
      | Issue 1.1: 23/11/2004: Hysterisis added to open/shut pressure - SW
      | Issue 1.2: 07/12/2004: Forced shut if isolated - SW
      | Issue 1.3: 28/10/2005: Added to FSP generic Library - DR
      | Issue 1.4: 9/12/2008: Fixed open for stability - SW
  note: Calculate pressure drop across coupling
  note: Check if coupling is open - hysteresis
  Abs : Abs  SaturateOnIntegerOverflow=on
  BBBrk : FuelSystemLibrary/BBBrk
  BBBrk1 : FuelSystemLibrary/BBBrk1
  BBSrcAvailOut1 : FuelSystemLibrary/BBSrcAvailOut
  BBSrcAvailOut2 : FuelSystemLibrary/BBSrcAvailOut
  Constant : Constant  Value=DiscreteSwitchOn
  Constant4 : Constant  Value=CouplingOnPressure
  Constant5 : Constant  Value=CouplingOffPressure
  Ideal Switch : WrightSolverLib/Ideal Switch  OnResistance=LinearCouplingResistance
  Logical Operator1 : Logic  Operator=OR  AllPortsSameDT=off
  Logical Operator2 : Logic  AllPortsSameDT=off
  Open/Shut : UnitDelay  SampleTime=FspSamplingPeriod
  PressTap1 : FuelSystemLibrary/PressTap
  PressTap2 : FuelSystemLibrary/PressTap
  Relational Operator : RelationalOperator  Operator=>  InputSameDT=on
  Sum : Sum  Inputs=|+-  SaturateOnIntegerOverflow=on
  Switch1 : Switch  Threshold=BoolThreshold  SaturateOnIntegerOverflow=on  InputSameDT=on
  Terminator : Terminator
  Terminator3 : Terminator
  1P : PMIOPort  Tag=PMCPort  Port=1  Side=Left
  2P : PMIOPort  Tag=PMCPort  Port=2  Side=Right
  1BB : PMIOPort  Tag=PMCPort  Port=3  Side=Left
  2BB : PMIOPort  Tag=PMCPort  Port=4  Side=Right
  wires:
  BBSrcAvailOut2/1 -> [End2Src]
  BBSrcAvailOut1/1 -> [End1Src]
  BBBrk1/1 -> BBSrcAvailOut2/1, BBBrk/1, BBSrcAvailOut1/1
  BBBrk/1 -> BBBrk1/1
  Sum/1 -> Abs/1  "PressureDrop"
  Logical Operator2/1 -> Open/Shut/1
  Relational Operator/1 -> Logical Operator2/1
  Logical Operator1/1 -> Logical Operator2/2
  [End2Src] -> Logical Operator1/2
  [End1Src] -> Logical Operator1/1
  Abs/1 -> Relational Operator/1
  [ValveOpen] -> Switch1/2
  Constant4/1 -> Switch1/3
  Constant5/1 -> Switch1/1
  Open/Shut/1 -> Terminator/1
  Switch1/1 -> Relational Operator/2
  [OutputPressure] -> Sum/2
  [InputPressure] -> Sum/1
  PressTap2/1 -> [OutputPressure]
  [ValveOpen] -> Ideal Switch/1
  PressTap1/1 -> [InputPressure]
  Constant/1 -> [ValveOpen]
  Ideal Switch/1 -> Terminator3/1
  connections:
  1BB/RConn1 -- BBBrk1/RConn1
  BBBrk/LConn1 -- 2BB/RConn1
  Ideal Switch/RConn1 -- PressTap2/LConn1
  PressTap2/RConn1 -- 2P/RConn1
  1P/RConn1 -- PressTap1/LConn1
  PressTap1/RConn1 -- Ideal Switch/LConn1

== system FuelSystemLibrary/GTZero ==
  note: GTZero
      |
      | Revision History -
      | Issue 1.0 - ?? - SW - Initial Issue
      | Issue 1.1 - 28th October 2005 - DR - Added to FSP Generic Library
  In : Inport
  Constant : Constant  Value=0
  Relational Operator : RelationalOperator  Operator=>  InputSameDT=on
  >0 : Outport
  wires:
  In/1 -> Relational Operator/1
  Relational Operator/1 -> >0/1
  Constant/1 -> Relational Operator/2

== system FuelSystemLibrary/InPlug ==
  note: InPlug
      |
      | Revision History -
      | Issue 1.0 - ?? - SW - Initial Issue
      | Issue 1.1 - 28th October 2005 - DR - Added to FSP Generic Library
  BBTerm : FuelSystemLibrary/BBTerm
  Constant1 : Constant  Value=InfiniteResistance
  LineSolver : WrightSolverLib/LineSolver
  Res : WrightSolverLib/Res
  Term : WrightSolverLib/Term
  Terminator3 : Terminator
  1P : PMIOPort  Tag=PMCPort  Port=1  Side=Right
  1BB : PMIOPort  Tag=PMCPort  Port=2  Side=Right
  wires:
  Constant1/1 -> Res/1
  Res/1 -> Terminator3/1
  connections:
  BBTerm/LConn1 -- 1BB/RConn1
  Res/RConn1 -- 1P/RConn1
  LineSolver/RConn1 -- Res/LConn1
  Term/RConn1 -- LineSolver/LConn1

== system FuelSystemLibrary/Inlet ==
  note: Inlet
      |
      | Revision History -
      | Issue 1.0 - ?? - SW - Initial Issue
      | Issue 1.1 - 28th October 2005 - DR - Added to FSP Generic Library
  note: Elevate the inlet pressure
      | due to head pressures.
  HeadPress : Inport
  PipeCovered : Inport  Port=2
  Error : Inport  Port=3
  FlowOverride : Inport  Port=4
  Constant8 : Constant  Value=FlowNoOverride
  Data Type Conversion1 : DataTypeConversion  OutDataTypeStr=double
  Ideal Switch1 : WrightSolverLib/Ideal Switch  OnResistance=TankInletResistance
  InsidePressTap : FuelSystemLibrary/PressTap
  OutsidePressTap : FuelSystemLibrary/PressTap
  S-Function : S-Function  FunctionName=InletControlBlockWrapper  EnableBusSupport=off
  Term : WrightSolverLib/Term
  Unit Delay : UnitDelay  SampleTime=-1
  Unit Delay1 : UnitDelay  SampleTime=-1
  V : WrightSolverLib/V
  1P : PMIOPort  Tag=PMCPort  Port=1  Side=Left
  InFlow : Outport
  wires:
  Unit Delay/1 -> Ideal Switch1/1
  Error/1 -> S-Function/5
  Unit Delay1/1 -> S-Function/6
  S-Function/2 -> Unit Delay1/1
  S-Function/1 -> Unit Delay/1
  [InFlow] -> InFlow/1
  [InFlow] -> S-Function/4
  [InsidePressure] -> S-Function/3
  [OutsidePressure] -> S-Function/2
  InsidePressTap/1 -> [InsidePressure]
  OutsidePressTap/1 -> [OutsidePressure]
  PipeCovered/1 -> Data Type Conversion1/1
  Ideal Switch1/1 -> [InFlow]
  HeadPress/1 -> V/1
  FlowOverride/1 -> V/3
  Constant8/1 -> V/2
  Data Type Conversion1/1 -> S-Function/1
  connections:
  Ideal Switch1/RConn1 -- InsidePressTap/LConn1
  Term/RConn1 -- V/LConn1
  V/RConn1 -- InsidePressTap/RConn1
  1P/RConn1 -- OutsidePressTap/LConn1
  OutsidePressTap/RConn1 -- Ideal Switch1/LConn1

== system FuelSystemLibrary/LTZero ==
  note: LTZero
      |
      | Revision History -
      | Issue 1.0 - ?? - SW - Initial Issue
      | Issue 1.1 - 28th October 2005 - DR - Added to FSP Generic Library
  In : Inport
  Constant : Constant  Value=0
  Relational Operator : RelationalOperator  Operator=<  InputSameDT=on
  <0 : Outport
  wires:
  In/1 -> Relational Operator/1
  Constant/1 -> Relational Operator/2
  Relational Operator/1 -> <0/1

== system FuelSystemLibrary/Mass ==
  note: Mass - Seperate Mass signal from Instrumentation signal
      |
      | Revision History -
      | Issue 1.0 - ?? - SW - Initial Issue
      | Issue 1.1 - 28th October 2005 - DR - Added to FSP Generic Library
  Inst : Inport
  Demux4 : Demux  Outputs=20
  Terminator{1..19} (19 alike) : Terminator
  Mass : Outport
  wires:
  Demux4/12 -> Terminator3/1  "HeadPress"
  Demux4/11 -> Terminator9/1  "CG_Lat"
  Demux4/10 -> Terminator8/1  "CG_Long"
  Demux4/9 -> Terminator7/1  "CG_Vert"
  Demux4/8 -> Terminator19/1  "BValue"
  Demux4/7 -> Terminator18/1  "AValue"
  Demux4/6 -> Terminator17/1  "Temp"
  Demux4/5 -> Terminator2/1  "InFlow"
  Demux4/4 -> Terminator1/1  "SurfaceHeight"
  Demux4/3 -> Terminator16/1  "Volume"
  Demux4/2 -> Mass/1  "Mass"
  Demux4/1 -> Terminator4/1  "MaxVolume"
  Inst/1 -> Demux4/1
  Demux4/15 -> Terminator5/1  "LatPos"
  Demux4/14 -> Terminator10/1  "LongPos"
  Demux4/13 -> Terminator6/1  "VertPos"
  Demux4/20 -> Terminator13/1  "Outlet2Height"
  Demux4/19 -> Terminator11/1  "Outlet1Height"
  Demux4/18 -> Terminator14/1  "Inlet3Height"
  Demux4/17 -> Terminator12/1  "Inlet2Height"
  Demux4/16 -> Terminator15/1  "Inlet1Height"

== system FuelSystemLibrary/MassV3 ==
  note: Mass - Seperate Mass signal from Instrumentation signal
      |
      | Revision History -
      | Issue 1.0 - 11th Oct 2012 - SW - Initial Issue
  note: Volume
  InstV3 : Inport
  Demux4 : Demux  Outputs=22
  Terminator{1..21} (21 alike) : Terminator
  Mass : Outport
  wires:
  Demux4/18 -> Terminator15/1  "Inlet3Height"
  Demux4/19 -> Terminator12/1  "Outlet1Height"
  Demux4/20 -> Terminator14/1  "Outlet2Height"
  Demux4/21 -> Terminator11/1  "Outlet1Height"
  Demux4/22 -> Terminator13/1  "Outlet2Height"
  Demux4/15 -> Terminator6/1  "LatPos"
  Demux4/16 -> Terminator10/1  "Inlet1Height"
  Demux4/17 -> Terminator5/1  "Inlet2Height"
  Demux4/1 -> Terminator4/1  "MaxVolume"
  Demux4/2 -> Mass/1  "Mass"
  Demux4/4 -> Terminator1/1  "SurfaceHeight"
  Demux4/5 -> Terminator2/1  "InFlow"
  Demux4/6 -> Terminator17/1  "Temp"
  Demux4/7 -> Terminator18/1  "AValue"
  Demux4/8 -> Terminator19/1  "BValue"
  Demux4/11 -> Terminator7/1  "CG_Lat"
  Demux4/12 -> Terminator8/1  "HeadPress"
  Demux4/13 -> Terminator9/1  "VertPos"
  Demux4/14 -> Terminator3/1  "LongPos"
  Demux4/3 -> Terminator16/1
  Demux4/9 -> Terminator20/1  "Dielectric"
  Demux4/10 -> Terminator21/1  "Density"
  InstV3/1 -> Demux4/1

== system FuelSystemLibrary/Meter ==
  note: Summing mechanism, with reset
      |
      | Uses crude rectangular integrator, for
      | commonality with Tank summing system
      |
      |
      | Revision History -
      | Issue 1.0 - ?? - SW - Initial Issue
      | Issue 1.1 - 28th October 2005 - DR - Added to FSP Generic Library
  Reset : Inport
  Sig : Inport  Port=2
  Constant10 : Constant  Value=TankNoReset
  PerSec2PerCycle : Gain  Gain=PerSec2PerCycle  OutDataTypeStr=Inherit: Same as input  ParamDataTypeStr=Inherit: Same as input
  Relational Operator2 : RelationalOperator  Operator===  InputSameDT=on
  Sum2 : Sum  Inputs=|++  SaturateOnIntegerOverflow=on
  Switch3 : Switch  Threshold=BoolThreshold  SaturateOnIntegerOverflow=on  InputSameDT=on
  Unit Delay : UnitDelay  SampleTime=FspSamplingPeriod
  Sum : Outport
  wires:
  Sig/1 -> PerSec2PerCycle/1
  Sum2/1 -> Unit Delay/1
  Unit Delay/1 -> Sum/1, Switch3/1
  PerSec2PerCycle/1 -> Sum2/2
  Reset/1 -> Switch3/3, Relational Operator2/2
  Constant10/1 -> Relational Operator2/1
  Relational Operator2/1 -> Switch3/2
  Switch3/1 -> Sum2/1

== system FuelSystemLibrary/MixStub ==
  BBNull : FuelSystemLibrary/BBNull
  Constant : Constant  Value=0
  Nul : Outport
  Zero : Outport  Port=2
  wires:
  Constant/1 -> Zero/1
  BBNull/1 -> Nul/1

== system FuelSystemLibrary/NEZero ==
  note: NEZero
      |
      | Revision History -
      | Issue 1.0 - ?? - SW - Initial Issue
      | Issue 1.1 - 28th October 2005 - DR - Added to FSP Generic Library
  In : Inport
  Constant : Constant  Value=0
  Relational Operator : RelationalOperator  Operator=~=  InputSameDT=on
  !=0 : Outport
  wires:
  In/1 -> Relational Operator/1
  Constant/1 -> Relational Operator/2
  Relational Operator/1 -> !=0/1

== system FuelSystemLibrary/NRV ==
  note: NRV: Simulation of Non Return Valve
      |
      | Revision History -
      | Issue 1.0 - ?? - SW - Initial Issue
      | Issue 1.1 - 28th October 2005 - DR - Added to FSP Generic Library and Forced to shut if no flow available (Note - from A380 FSP NRV2)
  note: No source available downstream,
      | no sink available upstream
  BBBrk : FuelSystemLibrary/BBBrk
  BBBrk1 : FuelSystemLibrary/BBBrk1
  BBSrcBrk : FuelSystemLibrary/BBSrcBrk
  Constant2 : Constant  Value=NonRetResistance
  Diode : WrightSolverLib/Diode
  SinkBrk : FuelSystemLibrary/BBSinkBrk
  Terminator3 : Terminator
  1P : PMIOPort  Tag=PMCPort  Port=1  Side=Left
  2P : PMIOPort  Tag=PMCPort  Port=2  Side=Right
  1BB : PMIOPort  Tag=PMCPort  Port=3  Side=Left
  2BB : PMIOPort  Tag=PMCPort  Port=4  Side=Right
  wires:
  BBSrcBrk/1 -> BBBrk1/1
  BBBrk/1 -> BBSrcBrk/1
  SinkBrk/1 -> BBBrk/1
  BBBrk1/1 -> SinkBrk/1
  Constant2/1 -> Diode/1
  Diode/1 -> Terminator3/1
  connections:
  BBBrk/LConn1 -- 2BB/RConn1
  1BB/RConn1 -- BBBrk1/RConn1
  Diode/RConn1 -- 2P/RConn1
  1P/RConn1 -- Diode/LConn1
